simulink model "IP_LQG_PCI6221"  (R2026a)
settings: Solver=ode45  StopTime=200  EnableMultiTasking=on
values from neighbouring files (symbols this model uses):
  A_aug = [A zeros(5,1) ... (first row only)    [IP_MACRO.m]
  ALPHA_MAX = 90 * pi/180    (= 1.57079632679)    [IP_MACRO.m]
  B_aug = [B; 0]    [IP_MACRO.m]
  BETA_MAX = 15 * pi/180    (= 0.261799387799)    [IP_MACRO.m]
  C_aug = [C zeros(2,1)]    [IP_MACRO.m]
  K = lqr(A_aug, B_aug, Qr, Rr)    [IP_MACRO.m]
  L_aug = [L ... (first row only)    [IP_MACRO.m]
  TIME_DELAY = 6    [IP_MACRO.m]
  Ts = 0.001    [IP_MACRO.m]
  V_MAX = 5    [IP_MACRO.m]
  V_MIN = -5    [IP_MACRO.m]
undefined symbols (not defined in the file or in its folder): National_Instruments, PCI
libraries: sldrtlib x3, simulink x2
settings Model: SimulationMode=external  ExtModeTrigDuration=100000  Creator=Alunos  LastModifiedBy=Tomas Teixeira
settings DebuggingCC: MergeDetectMultiDrivingBlocksExec=error
settings HardwareCC: ProdHWDeviceType=Intel->x86/Pentium  TargetIntDivRoundTo=Zero  TargetEndianess=LittleEndian  TargetHWDeviceType=Intel->x86/Pentium
settings RTWCC: SystemTargetFile=rtwin.tlc  TemplateMakefile=rtwin.tmf  RTWCompilerOptimization=on  Description=Simulink Desktop Real-Time
settings CodeAppCC: MaxIdLength=95.0
settings GRTTargetCC: ModelReferenceCompliant=off  ParMdlRefBuildCompliant=off  CompOptLevelCompliant=off  ConcurrentExecutionCompliant=off  CombineOutputUpdateFcns=off  MatFileLogging=off  MATLABClassNameForMDSCustomization=Simulink.SoftwareTarget.TargetSpecificTriggerConfigurationBase  CPPClassGenCompliant=off  GRTInterface=on
settings RTWinTargetCC: TargetPreCompLibLocation=C:\Program Files\MATLAB\R2015a\toolbox\sldrt\lib\win32

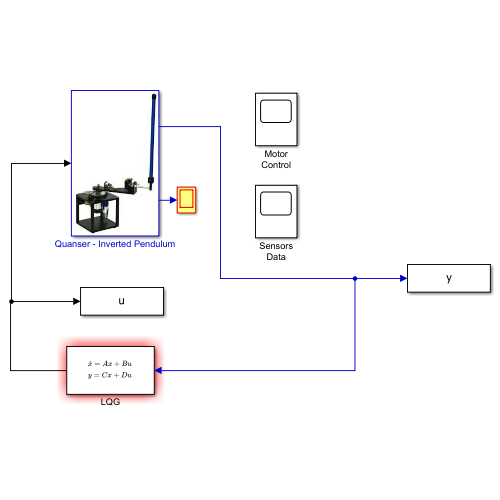
[thumbnail: Simulink's stored preview of the top-level diagram]
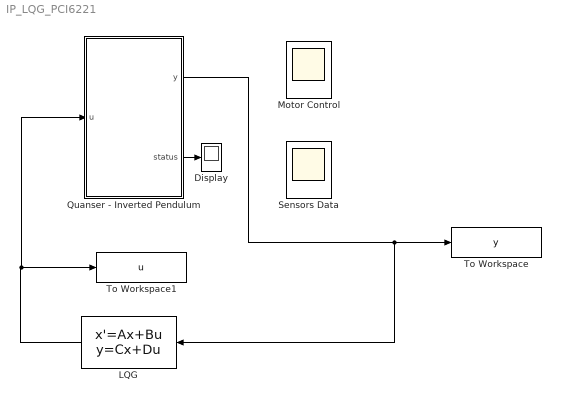
== system IP_LQG_PCI6221 ==
  Display : Display
  LQG : StateSpace  A=A_aug - B_aug * K - L_aug * C_aug  B=L_aug  C=-K  D=zeros(1,2)  InitialCondition=zeros(6,1)
  Motor Control : Scope
      settings: IsFloating=on  Floating=on  DataLoggingVariableName=ScopeData2
  Quanser - Inverted Pendulum : Subsystem
      mask Display: image('IP_QUANSER.jpg');
  Sensors Data : Scope
      settings: IsFloating=on  Floating=on  ActiveDisplayYMinimum=-3.1915926535897929  ActiveDisplayYMaximum=3.1915926535897929
  To Workspace : ToWorkspace  VariableName=y  SampleTime=-1
  To Workspace1 : ToWorkspace  VariableName=u  SampleTime=-1
  wires:
  Quanser - Inverted Pendulum/1(y) -> LQG/1, To Workspace/1
  Quanser - Inverted Pendulum/2(status) -> Display/1
  LQG/1 -> Quanser - Inverted Pendulum/1(u), To Workspace1/1

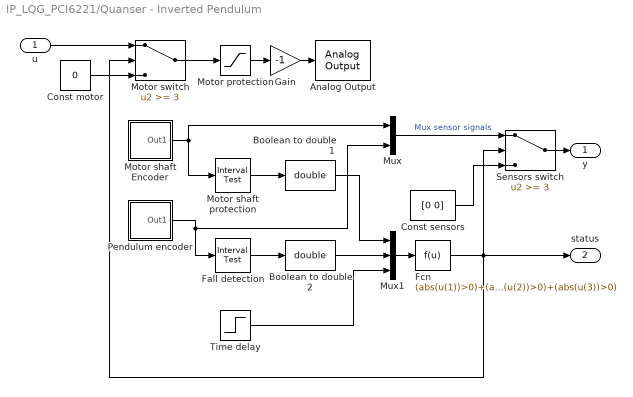
== system IP_LQG_PCI6221/Quanser - Inverted Pendulum ==
  u : Inport
  Analog Output : sldrtlib/Analog Output  SampleTime=Ts  MaxMissedTicks=10  ShowMissedTicks=off  YieldWhenWaiting=off  DrvName=National_Instruments/PCI-6221  DrvAddress=4294967295  DrvOptions=[0 0 0 2 2]  Channels=1  RangeMode=1  VoltRange=1  InitialValue=0  FinalValue=0
      settings: AttributesFormatString=National Instruments\nPCI-6221 [auto]
  Boolean to double 1 : DataTypeConversion  OutDataTypeStr=double  SaturateOnIntegerOverflow=off  RndMeth=Floor
  Boolean to double 2 : DataTypeConversion  OutDataTypeStr=double  SaturateOnIntegerOverflow=off  RndMeth=Floor
  Const motor : Constant  Value=0
  Const sensors : Constant  Value=[0 0]
  Fall detection : simulink/Logic and Bit Operations/Interval Test  IntervalClosedRight=on  uplimit=BETA_MAX  IntervalClosedLeft=on  lowlimit=-BETA_MAX  OutDataTypeStr=uint8
  Fcn : Fcn  Expr=(abs(u(1))>0)+(abs(u(2))>0)+(abs(u(3))>0)
  Gain : Gain  Gain=-1
  Motor protection : Saturate  UpperLimit=V_MAX  LowerLimit=V_MIN
  Motor shaft Encoder : Subsystem
  Motor shaft protection : simulink/Logic and Bit Operations/Interval Test  IntervalClosedRight=on  uplimit=ALPHA_MAX  IntervalClosedLeft=on  lowlimit=-ALPHA_MAX  OutDataTypeStr=uint8
  Motor switch : Switch  Threshold=3  SaturateOnIntegerOverflow=off  InputSameDT=off
  Mux : Mux  Inputs=2
  Mux1 : Mux  Inputs=3
  Pendulum encoder : Subsystem
  Sensors switch : Switch  Threshold=3  SaturateOnIntegerOverflow=off  InputSameDT=off
  Time delay : Step  Time=TIME_DELAY  SampleTime=0
  y : Outport
  status : Outport  Port=2
  wires:
  u/1 -> Motor switch/1
  Motor switch/1 -> Motor protection/1
  Const motor/1 -> Motor switch/3
  Motor shaft Encoder/1(Out1) -> Mux/1, Motor shaft protection/1
  Pendulum encoder/1(Out1) -> Fall detection/1, Mux/2
  Mux1/1 -> Fcn/1
  Fcn/1 -> Sensors switch/2, status/1, Motor switch/2
  Time delay/1 -> Mux1/3
  Fall detection/1 -> Boolean to double 2/1
  Boolean to double 2/1 -> Mux1/2
  Motor shaft protection/1 -> Boolean to double 1/1
  Boolean to double 1/1 -> Mux1/1
  Const sensors/1 -> Sensors switch/3
  Mux/1 -> Sensors switch/1  "Mux sensor signals"
  Sensors switch/1 -> y/1
  Gain/1 -> Analog Output/1
  Motor protection/1 -> Gain/1

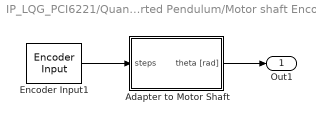
== system IP_LQG_PCI6221/Quanser - Inverted Pendulum/Motor shaft Encoder ==
  Adapter to Motor Shaft : Subsystem
  Encoder Input1 : sldrtlib/Encoder Input  SampleTime=Ts  MaxMissedTicks=inf  ShowMissedTicks=off  YieldWhenWaiting=off  DrvName=National_Instruments/PCI-6221  DrvAddress=4294967295  DrvOptions=[0 0 0 2 2]  Channels=1  QuadMode=3  IndexPulse=2  InputFilter=Inf  DataType=1
      settings: AttributesFormatString=National Instruments\nPCI-6221 [auto]
  Out1 : Outport
  wires:
  Encoder Input1/1 -> Adapter to Motor Shaft/1(steps)
  Adapter to Motor Shaft/1(theta [rad]) -> Out1/1

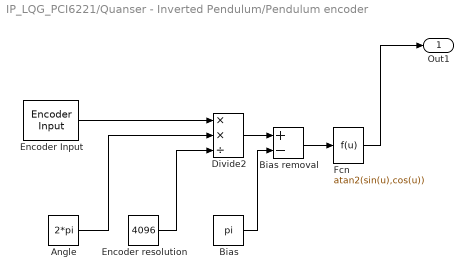
== system IP_LQG_PCI6221/Quanser - Inverted Pendulum/Pendulum encoder ==
  Angle : Constant  Value=2*pi
  Bias : Constant  Value=pi
  Bias removal : Sum  Inputs=+-
  Divide2 : Product  Inputs=**/
  Encoder resolution : Constant  Value=4096
  Encoder Input : sldrtlib/Encoder Input  SampleTime=Ts  MaxMissedTicks=inf  ShowMissedTicks=off  YieldWhenWaiting=off  DrvName=National_Instruments/PCI-6221  DrvAddress=4294967295  DrvOptions=[0 0 0 2 2]  Channels=2  QuadMode=3  IndexPulse=2  InputFilter=Inf  DataType=1
      settings: AttributesFormatString=National Instruments\nPCI-6221 [auto]
  Fcn : Fcn  Expr=atan2(sin(u),cos(u))
  Out1 : Outport
  wires:
  Bias/1 -> Bias removal/2
  Encoder resolution/1 -> Divide2/3
  Divide2/1 -> Bias removal/1
  Fcn/1 -> Out1/1
  Encoder Input/1 -> Divide2/1
  Bias removal/1 -> Fcn/1
  Angle/1 -> Divide2/2

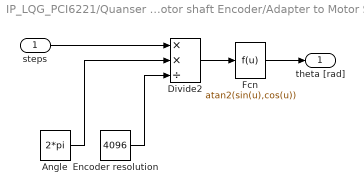
== system IP_LQG_PCI6221/Quanser - Inverted Pendulum/Motor shaft Encoder/Adapter to Motor Shaft ==
  steps : Inport
  Angle : Constant  Value=2*pi
  Divide2 : Product  Inputs=**/
  Encoder resolution : Constant  Value=4096
  Fcn : Fcn  Expr=atan2(sin(u),cos(u))
  theta [rad] : Outport
  wires:
  Angle/1 -> Divide2/2
  Encoder resolution/1 -> Divide2/3
  steps/1 -> Divide2/1
  Divide2/1 -> Fcn/1
  Fcn/1 -> theta [rad]/1
